simulink model "MyPCImages"  (Simulink 7.5)
settings: Solver=FixedStepDiscrete  StartTime=0.0  StopTime=d_data(end,1)  FixedStep=apSampleTime  RelTol=1e-3
InitFcn:
  | replayFlight
values from neighbouring files (symbols this model uses):
  apSampleTime = 0.01    [demoz2SlugsV5.m]
  D = y    [BarOrthog.m]
  R0 = single(Euler2DCMdeg( PHI_IC, THETA_IC, PSI_IC ))    [demoz2SlugsV5.m]
undefined symbols (not defined in the file or in its folder): accBiasRateLimit, accelXCutTemp, axTGain1, axTGain2, axTMean1, axTMean2, barAdjust, baroCutoff, baroCutTemp, baroOffset, baroScale, barTGain1, barTGain2, barTMean1, barTMean2, baseHeight, baseTemp, cubeAccelGain, cubeGyroGain, gaind, GS_location, gyroBiasRateLimit, Init_onlyOnce, Init_Reset, ISA_rho0, lapseRate, lowRateSensorCutoff, magMeanTemp, magOffset, magScale, magTempK, mainSensorCutoff, maxDynPressure, param_acc, param_mag, pitAdjust, pitCutTemp, pitotOffset, pitotScale, pitTGain1, pitTGain2, pitTMean1, pitTMean2, polesd, powerOffset, powerScale, pressureSensorCutoff, T, tempOffset, tempScale, vzCutoff, xCutoff, yCutoff, zCutoff, zerosd
libraries: simulink x11, aerolibconvert2 x9, SLUGS_Library x6, aerolibutil x3, dspmtrx3 x3, dsPICdrivers x1
(part 4 of 4)

== system MyPCImages/Sensor Data/Sensor Suite/Low Pass Filtering,Temperature Compensation and Calibration/Baro Altimeter/Zero Out Height ==
  Base Height : Inport  OutDataType=sfix(16)  OutScaling=2^0
  Computed Height : Inport  Port=2  OutDataType=sfix(16)  OutScaling=2^0
  Enable : EnablePort
  Integer Delay : simulink/Discrete/Integer Delay  vinit=0  samptime=.01  NumDelays=1
  Sum : Sum  Inputs=|+-  OutDataTypeMode=single  OutDataType=sfix(16)  OutScaling=2^0  OutDataTypeStr=single
  Height Offset : Outport  OutDataType=sfix(16)  OutScaling=2^0
  wires:
  Base Height/1 -> Sum/1
  Integer Delay/1 -> Sum/2
  Sum/1 -> Height Offset/1
  Computed Height/1 -> Integer Delay/1

== system MyPCImages/Sensor Data/Sensor Suite/Low Pass Filtering,Temperature Compensation and Calibration/Temp Compensate Accel X1/Hi Temp Compensation2 ==
  Raw : Inport  OutDataType=sfix(16)  OutScaling=2^0
  Temp Raw : Inport  Port=2  OutDataType=sfix(16)  OutScaling=2^0
  Enable : EnablePort
  Divide1 : Product  OutDataTypeMode=single  OutDataType=sfix(16)  OutScaling=2^-10  OutDataTypeStr=single
  Mean Temperature for Calibration : Constant  Value=tempMean  OutDataTypeMode=single  OutDataType=sfix(16)  OutScaling=2^0  OutDataTypeStr=single
  Sum1 : Sum  Inputs=|+-  OutDataTypeMode=single  OutDataType=sfix(16)  OutScaling=2^0  OutDataTypeStr=single
  Sum2 : Sum  Inputs=|+-  OutDataTypeMode=single  OutDataType=sfix(16)  OutScaling=2^0  OutDataTypeStr=single
  gains : Constant  Value=alpha  OutDataTypeMode=single  OutDataType=sfix(16)  OutScaling=2^0  OutDataTypeStr=single
  Comp : Outport  OutDataType=sfix(16)  OutScaling=2^0
  wires:
  Sum2/1 -> Comp/1
  Divide1/1 -> Sum2/2
  gains/1 -> Divide1/1
  Sum1/1 -> Divide1/2
  Temp Raw/1 -> Sum1/1
  Raw/1 -> Sum2/1
  Mean Temperature for Calibration/1 -> Sum1/2

== system MyPCImages/Sensor Data/Sensor Suite/Low Pass Filtering,Temperature Compensation and Calibration/Temp Compensate Accel X1/Lo Temp Compensation ==
  Raw : Inport  OutDataType=sfix(16)  OutScaling=2^0
  Temp Raw : Inport  Port=2  OutDataType=sfix(16)  OutScaling=2^0
  Enable : EnablePort
  Add : Sum  OutDataTypeMode=single  OutDataType=sfix(16)  OutScaling=2^-10  OutDataTypeStr=single
  Constant : Constant  Value=pitAdjust  OutDataTypeMode=single  OutDataType=sfix(16)  OutScaling=2^0  OutDataTypeStr=single
  Divide1 : Product  OutDataTypeMode=single  OutDataType=sfix(16)  OutScaling=2^-10  OutDataTypeStr=single
  Mean Temperature for Calibration : Constant  Value=tempMean  OutDataTypeMode=single  OutDataType=sfix(16)  OutScaling=2^0  OutDataTypeStr=single
  Sum1 : Sum  Inputs=|+-  OutDataTypeMode=single  OutDataType=sfix(16)  OutScaling=2^0  OutDataTypeStr=single
  Sum2 : Sum  Inputs=|+-  OutDataTypeMode=single  OutDataType=sfix(16)  OutScaling=2^0  OutDataTypeStr=single
  gains : Constant  Value=alpha  OutDataTypeMode=single  OutDataType=sfix(16)  OutScaling=2^0  OutDataTypeStr=single
  Comp : Outport  OutDataType=sfix(16)  OutScaling=2^0
  wires:
  Mean Temperature for Calibration/1 -> Sum1/2
  Raw/1 -> Sum2/1
  Temp Raw/1 -> Sum1/1
  Sum1/1 -> Divide1/2
  gains/1 -> Divide1/1
  Divide1/1 -> Sum2/2
  Sum2/1 -> Add/1
  Constant/1 -> Add/2
  Add/1 -> Comp/1

== system MyPCImages/Sensor Data/Sensor Suite/Low Pass Filtering,Temperature Compensation and Calibration/Temp Compensate Baro/Hi Temp Compensation ==
  Raw : Inport  OutDataType=sfix(16)  OutScaling=2^0
  Temp Raw : Inport  Port=2  OutDataType=sfix(16)  OutScaling=2^0
  Enable : EnablePort
  Add : Sum  OutDataTypeMode=single  OutDataType=sfix(16)  OutScaling=2^-10  OutDataTypeStr=single
  Constant : Constant  Value=barAdjust  OutDataTypeMode=single  OutDataType=sfix(16)  OutScaling=2^0  OutDataTypeStr=single
  Divide1 : Product  OutDataTypeMode=single  OutDataType=sfix(16)  OutScaling=2^-10  OutDataTypeStr=single
  Mean Temperature for Calibration : Constant  Value=tempMean  OutDataTypeMode=single  OutDataType=sfix(16)  OutScaling=2^0  OutDataTypeStr=single
  Sum1 : Sum  Inputs=|+-  OutDataTypeMode=single  OutDataType=sfix(16)  OutScaling=2^0  OutDataTypeStr=single
  Sum2 : Sum  Inputs=|+-  OutDataTypeMode=single  OutDataType=sfix(16)  OutScaling=2^0  OutDataTypeStr=single
  gains : Constant  Value=alpha  OutDataTypeMode=single  OutDataType=sfix(16)  OutScaling=2^0  OutDataTypeStr=single
  Comp : Outport  OutDataType=sfix(16)  OutScaling=2^0
  wires:
  Mean Temperature for Calibration/1 -> Sum1/2
  Raw/1 -> Sum2/1
  Temp Raw/1 -> Sum1/1
  Sum1/1 -> Divide1/2
  gains/1 -> Divide1/1
  Divide1/1 -> Sum2/2
  Constant/1 -> Add/1
  Add/1 -> Comp/1
  Sum2/1 -> Add/2

== system MyPCImages/Sensor Data/Sensor Suite/Low Pass Filtering,Temperature Compensation and Calibration/Temp Compensate Baro/Lo Temp Compensation ==
  Raw : Inport  OutDataType=sfix(16)  OutScaling=2^0
  Temp Raw : Inport  Port=2  OutDataType=sfix(16)  OutScaling=2^0
  Enable : EnablePort
  Divide1 : Product  OutDataTypeMode=single  OutDataType=sfix(16)  OutScaling=2^-10  OutDataTypeStr=single
  Mean Temperature for Calibration : Constant  Value=tempMean  OutDataTypeMode=single  OutDataType=sfix(16)  OutScaling=2^0  OutDataTypeStr=single
  Sum1 : Sum  Inputs=|+-  OutDataTypeMode=single  OutDataType=sfix(16)  OutScaling=2^0  OutDataTypeStr=single
  Sum2 : Sum  Inputs=|+-  OutDataTypeMode=single  OutDataType=sfix(16)  OutScaling=2^0  OutDataTypeStr=single
  gains : Constant  Value=alpha  OutDataTypeMode=single  OutDataType=sfix(16)  OutScaling=2^0  OutDataTypeStr=single
  Comp : Outport  OutDataType=sfix(16)  OutScaling=2^0
  wires:
  Sum2/1 -> Comp/1
  Divide1/1 -> Sum2/2
  gains/1 -> Divide1/1
  Sum1/1 -> Divide1/2
  Temp Raw/1 -> Sum1/1
  Raw/1 -> Sum2/1
  Mean Temperature for Calibration/1 -> Sum1/2

== system MyPCImages/Sensor Data/Sensor Suite/Low Pass Filtering,Temperature Compensation and Calibration/ValidateMags/Hold if Outlier ==
  In1 : Inport  OutDataType=sfix(16)  OutScaling=2^0
  Enable : EnablePort
  Out1 : Outport  OutDataType=sfix(16)  OutScaling=2^0  OutputWhenDisabled=reset  InitialOutput=[0 0 0]
  wires:
  In1/1 -> Out1/1

== system MyPCImages/Sensor Data/Sensor Suite/Low Pass Filtering,Temperature Compensation and Calibration/ValidateMags/Monitor Norm ==
  Mags : Inport  OutDataType=sfix(16)  OutScaling=2^0
  0.7 < Norm < 1.5 : Subsystem
  Norm : Subsystem  AncestorBlock=SLUGS_Library/Navigation/Norm
  Enable : Outport  OutDataType=sfix(16)  OutScaling=2^0
  wires:
  Mags/1 -> Norm/1(Vector)
  0.7 < Norm < 1.5/1(flag) -> Enable/1
  Norm/1(Norm) -> 0.7 < Norm < 1.5/1(norm)

== system MyPCImages/Position and Attitude Filter/Position Filter/BlendPosVel/2 FIlter Blend/1D Filter/Filter2 ==
  In1 : Inport  OutDataType=sfix(16)  OutScaling=2^0
  Discrete Zero-Pole : DiscreteZeroPole  Zeros=zerosd  Poles=polesd  Gain=gaind  SampleTime=SampleTime
  Out1 : Outport  OutDataType=sfix(16)  OutScaling=2^0
  wires:
  Discrete Zero-Pole/1 -> Out1/1
  In1/1 -> Discrete Zero-Pole/1

== system MyPCImages/Position and Attitude Filter/Position Filter/BlendPosVel/2 FIlter Blend/1D Filter1/Filter2 ==
  In1 : Inport  OutDataType=sfix(16)  OutScaling=2^0
  Discrete Zero-Pole : DiscreteZeroPole  Zeros=zerosd  Poles=polesd  Gain=gaind  SampleTime=SampleTime
  Out1 : Outport  OutDataType=sfix(16)  OutScaling=2^0
  wires:
  In1/1 -> Discrete Zero-Pole/1
  Discrete Zero-Pole/1 -> Out1/1

== system MyPCImages/Position and Attitude Filter/Position Filter/BlendPosVel/CompFiltRate/1D Filter1/Filter2 ==
  In1 : Inport  OutDataType=sfix(16)  OutScaling=2^0
  Discrete Zero-Pole : DiscreteZeroPole  Zeros=zerosd  Poles=polesd  Gain=gaind  SampleTime=SampleTime
  Out1 : Outport  OutDataType=sfix(16)  OutScaling=2^0
  wires:
  In1/1 -> Discrete Zero-Pole/1
  Discrete Zero-Pole/1 -> Out1/1

== system MyPCImages/Position and Attitude Filter/Position Filter/BlendPosVel/CompFiltRate1/1D Filter1/Filter2 ==
  In1 : Inport  OutDataType=sfix(16)  OutScaling=2^0
  Discrete Zero-Pole : DiscreteZeroPole  Zeros=zerosd  Poles=polesd  Gain=gaind  SampleTime=SampleTime
  Out1 : Outport  OutDataType=sfix(16)  OutScaling=2^0
  wires:
  In1/1 -> Discrete Zero-Pole/1
  Discrete Zero-Pole/1 -> Out1/1

== system MyPCImages/Position and Attitude Filter/Position Filter/BlendPosVel/CompRateOnly/1D Filter1/Filter2 ==
  In1 : Inport  OutDataType=sfix(16)  OutScaling=2^0
  Discrete Zero-Pole : DiscreteZeroPole  Zeros=zerosd  Poles=polesd  Gain=gaind  SampleTime=SampleTime
  Out1 : Outport  OutDataType=sfix(16)  OutScaling=2^0
  wires:
  In1/1 -> Discrete Zero-Pole/1
  Discrete Zero-Pole/1 -> Out1/1

== system MyPCImages/Sensor Data/Sensor Suite/Low Pass Filtering,Temperature Compensation and Calibration/Baro Altimeter/Initial Baro Bias/Low Pass8 ==
  In1 : Inport  OutDataType=sfix(16)  OutScaling=2^0
  Discrete Zero-Pole : DiscreteZeroPole  Zeros=zerosd  Poles=polesd  Gain=gaind  SampleTime=SampleTime
  Out1 : Outport  OutDataType=sfix(16)  OutScaling=2^0
  wires:
  Discrete Zero-Pole/1 -> Out1/1
  In1/1 -> Discrete Zero-Pole/1

== system MyPCImages/Sensor Data/Sensor Suite/Low Pass Filtering,Temperature Compensation and Calibration/ValidateMags/Monitor Norm/0.7 < Norm < 1.5 ==
  norm : Inport  OutDataType=sfix(16)  OutScaling=2^0
  Compare To Constant : simulink/Logic and Bit Operations/Compare To Constant  SystemSampleTime=-1  relop=>  const=0.5  LogicOutDataTypeMode=uint8  ZeroCross=off
  Compare To Constant1 : simulink/Logic and Bit Operations/Compare To Constant  SystemSampleTime=-1  relop=<  const=1.6  LogicOutDataTypeMode=uint8  ZeroCross=off
  Logical Operator : Logic  AllPortsSameDT=off  OutDataTypeMode=boolean  OutDataTypeStr=boolean
  flag : Outport  OutDataType=sfix(16)  OutScaling=2^0
  wires:
  Logical Operator/1 -> flag/1
  norm/1 -> Compare To Constant1/1, Compare To Constant/1
  Compare To Constant/1 -> Logical Operator/1
  Compare To Constant1/1 -> Logical Operator/2

== system MyPCImages/Sensor Data/Sensor Suite/Low Pass Filtering,Temperature Compensation and Calibration/ValidateMags/Monitor Norm/Norm ==
  Vector : Inport  OutDataType=sfix(16)  OutScaling=2^0
  Subsystem1 : Subsystem  AncestorBlock=SLUGS_Library/Subsystem1
  Subsystem3 : Subsystem  AncestorBlock=SLUGS_Library/Subsystem3
  Norm : Outport  OutDataType=sfix(16)  OutScaling=2^0
  wires:
  Subsystem3/1(x dot y) -> Subsystem1/1(x)
  Vector/1 -> Subsystem3/2(y), Subsystem3/1(x)
  Subsystem1/1(sqrt(x)) -> Norm/1

== system MyPCImages/Sensor Data/Sensor Suite/Low Pass Filtering,Temperature Compensation and Calibration/ValidateMags/Monitor Norm/Norm/Subsystem1 ==
  x : Inport  OutDataType=sfix(16)  OutScaling=2^0
  C Function Call : dsPICdrivers/OTHERS/C Function Call  Tag=dsPIC_dsPIC_CFunctionCall  FctUpdate=Output Function  fctName='mySqrt'  INPUT_SIZE=1  INPUT1=real32  INPUT2=--  INPUT3=--  OUTPUT_SIZE=1  OUTPUT1=real32  SampleTime=-1  InputType=[ 7 ]  OutputType=[ 7 ]  FctDeclaration=extern real32_T mySqrt(real32_T u1);  FctCall=%y1 = mySqrt(%u1);  OrderingInOutPopup=None  FctStart=None  FctStart_Name=Init_onlyOnce  FctStart_Declaration=inline extern void Init_onlyOnce();  FctStart_Call=Init_onlyOnce();  FctInit=None  FctInit_Name=Init_Reset  FctInit_Declaration=inline extern void Init_Reset();  FctInit_Call=Init_Reset();  PinDigitalInput=[]  PinDigitalOutput=[]  AnalogueInput=[]
  negprotect : Stateflow chart  TreatAsAtomicUnit=on
  sqrt(x) : Outport  OutDataType=sfix(16)  OutScaling=2^0
  wires:
  C Function Call/1 -> sqrt(x)/1
  negprotect/1(zpVal) -> C Function Call/1
  x/1 -> negprotect/1(val)

== system MyPCImages/Sensor Data/Sensor Suite/Low Pass Filtering,Temperature Compensation and Calibration/ValidateMags/Monitor Norm/Norm/Subsystem3 ==
  x : Inport  OutDataType=sfix(16)  OutScaling=2^0
  y : Inport  Port=2  OutDataType=sfix(16)  OutScaling=2^0
  Embedded MATLAB Function : Stateflow chart  TreatAsAtomicUnit=on
  x dot y : Outport  OutDataType=sfix(16)  OutScaling=2^0
  wires:
  y/1 -> Embedded MATLAB Function/2(y)
  x/1 -> Embedded MATLAB Function/1(x)
  Embedded MATLAB Function/1(xDoty) -> x dot y/1

== matlab function Sensor Data/Sensor Suite/Low Pass Filtering,Temperature Compensation and Calibration/Tustin Lowpass, Auto Initial Condition2/Embedded MATLAB Function ==
  data: u input double; y output double; T input double; f input double
function y = fcn(u,T,f)
% This block supports an embeddable subset of the MATLAB language.
% See the help menu for details. 

persistent a
persistent b
persistent y_km1
persistent u_km1
if isempty(a)
    %tf = [T*omega/(2+T*omega) T*omega/(2+T*omega)],[1 (T*omega-2)/(T*omega+2)]
    %tf = [a a],[1 -b]
    omega = 2*pi*f;
    a=T*omega/(2+T*omega);
    b=-(T*omega-2)/(T*omega+2);
    y_km1=u;
    u_km1=u;
end

y = a*(u+u_km1)+b*y_km1;
y_km1=y;
u_km1=u;

== matlab function Sensor Data/Sensor Suite/Low Pass Filtering,Temperature Compensation and Calibration/Tustin Lowpass, Auto Initial Condition3/Embedded MATLAB Function ==
  data: u input double; y output double; T input double; f input double
function y = fcn(u,T,f)
% This block supports an embeddable subset of the MATLAB language.
% See the help menu for details. 

persistent a
persistent b
persistent y_km1
persistent u_km1
if isempty(a)
    %tf = [T*omega/(2+T*omega) T*omega/(2+T*omega)],[1 (T*omega-2)/(T*omega+2)]
    %tf = [a a],[1 -b]
    omega = 2*pi*f;
    a=T*omega/(2+T*omega);
    b=-(T*omega-2)/(T*omega+2);
    y_km1=u;
    u_km1=u;
end

y = a*(u+u_km1)+b*y_km1;
y_km1=y;
u_km1=u;

== matlab function Sensor Data/Sensor Suite/Low Pass Filtering,Temperature Compensation and Calibration/3D Tustin Lowpass, Auto Initial Condition/Embedded MATLAB Function ==
  data: u input double; y output double; T input double; f input double
function y = fcn(u,T,f)
% This block supports an embeddable subset of the MATLAB language.
% See the help menu for details. 

persistent a
persistent b
persistent y_km1
persistent u_km1
if isempty(a)
    %tf = [T*omega/(2+T*omega) T*omega/(2+T*omega)],[1 (T*omega-2)/(T*omega+2)]
    %tf = [a a],[1 -b]
    omega = 2*pi*f;
    a=T*omega/(2+T*omega);
    b=-(T*omega-2)/(T*omega+2);
    y_km1=u;
    u_km1=u;
end

y = a*(u+u_km1)+b*y_km1;
y_km1=y;
u_km1=u;

== matlab function Sensor Data/Sensor Suite/Low Pass Filtering,Temperature Compensation and Calibration/3D Tustin Lowpass, Auto Initial Condition/Embedded MATLAB Function1 ==
  data: u input double; y output double; T input double; f input double
function y = fcn(u,T,f)
% This block supports an embeddable subset of the MATLAB language.
% See the help menu for details. 

persistent a
persistent b
persistent y_km1
persistent u_km1
if isempty(a)
    %tf = [T*omega/(2+T*omega) T*omega/(2+T*omega)],[1 (T*omega-2)/(T*omega+2)]
    %tf = [a a],[1 -b]
    omega = 2*pi*f;
    a=T*omega/(2+T*omega);
    b=-(T*omega-2)/(T*omega+2);
    y_km1=u;
    u_km1=u;
end

y = a*(u+u_km1)+b*y_km1;
y_km1=y;
u_km1=u;

== matlab function Sensor Data/Sensor Suite/Low Pass Filtering,Temperature Compensation and Calibration/3D Tustin Lowpass, Auto Initial Condition/myMux Fun ==
  data: u1 input double; y output double; u2 input double; u3 input double
function y = myMux3(u1, u2, u3)
% This block supports an embeddable subset of the MATLAB language.
% See the help menu for details. 

y = [u1(1); u2(1); u3(1)];

== matlab function Sensor Data/Sensor Suite/Low Pass Filtering,Temperature Compensation and Calibration/Tustin Lowpass, Auto Initial Condition4/Embedded MATLAB Function ==
  data: u input double; y output double; T input double; f input double
function y = fcn(u,T,f)
% This block supports an embeddable subset of the MATLAB language.
% See the help menu for details. 

persistent a
persistent b
persistent y_km1
persistent u_km1
if isempty(a)
    %tf = [T*omega/(2+T*omega) T*omega/(2+T*omega)],[1 (T*omega-2)/(T*omega+2)]
    %tf = [a a],[1 -b]
    omega = 2*pi*f;
    a=T*omega/(2+T*omega);
    b=-(T*omega-2)/(T*omega+2);
    y_km1=u;
    u_km1=u;
end

y = a*(u+u_km1)+b*y_km1;
y_km1=y;
u_km1=u;

== matlab function Position and Attitude Filter/Attitude Complimentary Filter COG/3D Filter/myMux Fun1 ==
  data: u1 input double; y output double; u2 input double; u3 input double
function y = myMux(u1, u2, u3)
% This block supports an embeddable subset of the MATLAB language.
% See the help menu for details. 

y = [u1(1); u2(1); u3(1)];

== matlab function Sensor Data/Sensor Suite/Low Pass Filtering,Temperature Compensation and Calibration/Baro Altimeter/Enables/Disables the Computation of initial Baro Bias ==
  data: tOut output double
function tOut = getTIni

persistent aveCount;
persistent tIni;

if isempty(aveCount)
    aveCount =1;
    tIni = 1;
end;

if aveCount < 2500
    aveCount = aveCount + 1;
end

if aveCount == 2500
    tIni =0;
    aveCount = aveCount + 1;
end

tOut = tIni;

%if aveCount > 500
%    tIni = 0;
%end

% if isempty(aveCount)
%     aveCount =1;
%     initBias = [0.0 0.0 0.0]';
% end;
%     
% if (aveCount<10)
%     initBias = initBias+ Raw;
%     bias = initBias/aveCount;
%     aveCount = aveCount +1;
% end;
% 
% if (aveCount == 10)
%     initBias = initBias/(aveCount-1);
%     aveCount = 100;
% end;
% 
% if (aveCount == 100)
%     bias = initBias;
% end;

== matlab function Position and Attitude Filter/Attitude Complimentary Filter COG/Embedded MATLAB Function ==
  data: u input double; y output double
function y = TwoPi(u)
% This block supports an embeddable subset of the MATLAB language.
% See the help menu for details. 

if ( u < 0 )
    y = u + 2*pi;
else
    y = u;
end

== matlab function Sensor Data/Sensor Suite/Low Pass Filtering,Temperature Compensation and Calibration/3D Tustin Lowpass, Auto Initial Condition/Embedded MATLAB Function2 ==
  data: u input double; y output double; T input double; f input double
function y = fcn(u,T,f)
% This block supports an embeddable subset of the MATLAB language.
% See the help menu for details. 

persistent a
persistent b
persistent y_km1
persistent u_km1
if isempty(a)
    %tf = [T*omega/(2+T*omega) T*omega/(2+T*omega)],[1 (T*omega-2)/(T*omega+2)]
    %tf = [a a],[1 -b]
    omega = 2*pi*f;
    a=T*omega/(2+T*omega);
    b=-(T*omega-2)/(T*omega+2);
    y_km1=u;
    u_km1=u;
end

y = a*(u+u_km1)+b*y_km1;
y_km1=y;
u_km1=u;

== matlab function Sensor Data/Sensor Suite/Cube Signal Cond/3D Tustin Lowpass, Auto Initial Condition/Embedded MATLAB Function ==
  data: u input double; y output double; T input double; f input double
function y = fcn(u,T,f)
% This block supports an embeddable subset of the MATLAB language.
% See the help menu for details. 

persistent a
persistent b
persistent y_km1
persistent u_km1
if isempty(a)
    %tf = [T*omega/(2+T*omega) T*omega/(2+T*omega)],[1 (T*omega-2)/(T*omega+2)]
    %tf = [a a],[1 -b]
    omega = 2*pi*f;
    a=T*omega/(2+T*omega);
    b=-(T*omega-2)/(T*omega+2);
    y_km1=u;
    u_km1=u;
end

y = a*(u+u_km1)+b*y_km1;
y_km1=y;
u_km1=u;

== matlab function Sensor Data/Sensor Suite/Low Pass Filtering,Temperature Compensation and Calibration/Tustin Lowpass, Auto Initial Condition1/Embedded MATLAB Function ==
  data: u input double; y output double; T input double; f input double
function y = fcn(u,T,f)
% This block supports an embeddable subset of the MATLAB language.
% See the help menu for details. 

persistent a
persistent b
persistent y_km1
persistent u_km1
if isempty(a)
    %tf = [T*omega/(2+T*omega) T*omega/(2+T*omega)],[1 (T*omega-2)/(T*omega+2)]
    %tf = [a a],[1 -b]
    omega = 2*pi*f;
    a=T*omega/(2+T*omega);
    b=-(T*omega-2)/(T*omega+2);
    y_km1=u;
    u_km1=u;
end

y = a*(u+u_km1)+b*y_km1;
y_km1=y;
u_km1=u;

== matlab function Position and Attitude Filter/Attitude Complimentary Filter COG/myMux Fun1 ==
  data: u1 input double; y output double; u2 input double; u3 input double
function y = myMux3(u1, u2, u3)
% This block supports an embeddable subset of the MATLAB language.
% See the help menu for details. 

y = [u1(1); u2(1); u3(1)];

== matlab function Sensor Data/Sensor Suite/Low Pass Filtering,Temperature Compensation and Calibration/ValidateMags/Monitor Norm/Norm/Subsystem3/Embedded MATLAB Function ==
  data: x input double; y input double; xDoty output double
function xDoty = myDot(x,y)
% This block supports an embeddable subset of the MATLAB language.
% See the help menu for details. 

xDoty = x(1)*y(1) + x(2)*y(2) + x(3)*y(3);

== matlab function Sensor Data/Sensor Suite/Cube Signal Cond/3D Tustin Lowpass, Auto Initial Condition/Embedded MATLAB Function1 ==
  data: u input double; y output double; T input double; f input double
function y = fcn(u,T,f)
% This block supports an embeddable subset of the MATLAB language.
% See the help menu for details. 

persistent a
persistent b
persistent y_km1
persistent u_km1
if isempty(a)
    %tf = [T*omega/(2+T*omega) T*omega/(2+T*omega)],[1 (T*omega-2)/(T*omega+2)]
    %tf = [a a],[1 -b]
    omega = 2*pi*f;
    a=T*omega/(2+T*omega);
    b=-(T*omega-2)/(T*omega+2);
    y_km1=u;
    u_km1=u;
end

y = a*(u+u_km1)+b*y_km1;
y_km1=y;
u_km1=u;

== matlab function Sensor Data/Sensor Suite/Low Pass Filtering,Temperature Compensation and Calibration/ValidateMags/Monitor Norm/Norm/Subsystem1/negprotect ==
  data: val input double; zpVal output double
function zpVal = negProt(val)
% This block supports an embeddable subset of the MATLAB language.
% See the help menu for details. 

if val >= single(0.001)
    zpVal = val;
else
    zpVal = single(0.001);
end

== matlab function Position and Attitude Filter/Position Filter/BlendPosVel/3D Filter/myMux Fun1 ==
  data: u1 input double; y output double; u2 input double; u3 input double
function y = myMux(u1, u2, u3)
% This block supports an embeddable subset of the MATLAB language.
% See the help menu for details. 

y = [u1(1); u2(1); u3(1)];

== matlab function Sensor Data/Sensor Suite/Cube Signal Cond/3D Tustin Lowpass, Auto Initial Condition/Embedded MATLAB Function2 ==
  data: u input double; y output double; T input double; f input double
function y = fcn(u,T,f)
% This block supports an embeddable subset of the MATLAB language.
% See the help menu for details. 

persistent a
persistent b
persistent y_km1
persistent u_km1
if isempty(a)
    %tf = [T*omega/(2+T*omega) T*omega/(2+T*omega)],[1 (T*omega-2)/(T*omega+2)]
    %tf = [a a],[1 -b]
    omega = 2*pi*f;
    a=T*omega/(2+T*omega);
    b=-(T*omega-2)/(T*omega+2);
    y_km1=u;
    u_km1=u;
end

y = a*(u+u_km1)+b*y_km1;
y_km1=y;
u_km1=u;

== matlab function Sensor Data/Sensor Suite/If no HIL then Read all the Sensors/myMux Fun4 ==
  data: u1 input double; y output double; u2 input double; u3 input double; u4 input double; u5 input double; u6 input double; u7 input double; u8 input double; u9 input double; u10 input double; u11 input double; u12 input double; u13 input double
function y = sensMux(u1, u2,u3,u4,u5,u6,u7,u8, u9, u10, u11, u12, u13)
% This block supports an embeddable subset of the MATLAB language.
% See the help menu for details. 

y = [u1(1); u2(1); u3(1); u4(1); u5(1); u6(1); u7(1); u8(1); u9(1); u10(1); u11(1); u12(1); u13(1)];

== matlab function Sensor Data/Sensor Suite/Cube Signal Cond/3D Tustin Lowpass, Auto Initial Condition/myMux Fun ==
  data: u1 input double; y output double; u2 input double; u3 input double
function y = myMux3(u1, u2, u3)
% This block supports an embeddable subset of the MATLAB language.
% See the help menu for details. 

y = [u1(1); u2(1); u3(1)];

== matlab function Sensor Data/Sensor Suite/Low Pass Filtering,Temperature Compensation and Calibration/Ellipse Correction/myMux Fun3 ==
  data: u1 input double; y output double; u2 input double; u3 input double
function y = myMux(u1, u2, u3)
% This block supports an embeddable subset of the MATLAB language.
% See the help menu for details. 

y = [u1(1); u2(1); u3(1)];

== matlab function Sensor Data/Sensor Suite/Cube Signal Cond/Ellipse Correction/myMux Fun3 ==
  data: u1 input double; y output double; u2 input double; u3 input double
function y = myMux(u1, u2, u3)
% This block supports an embeddable subset of the MATLAB language.
% See the help menu for details. 

y = [u1(1); u2(1); u3(1)];

== matlab function Position and Attitude Filter/Position Filter/BlendPosVel/Embedded MATLAB Function1 ==
  data: u input double size=1; y output double size=1; NewGPS input double size=1; apSampleTime parameter double size=1
function y = RateAid(u,NewGPS,apSampleTime)
persistent LastU;
persistent TimeSinceLast;
persistent NGPS;
persistent rate;
persistent OldRate;

if (isempty(LastU))
    LastU = single(0.);
    TimeSinceLast = single(0);
    NGPS = single(0);
    rate = single(0);
    OldRate = single(0);
end

if (NewGPS)
    if ( NGPS ~= 0 )
        OldRate = rate;
        rate = single((u - LastU)/TimeSinceLast);
        TimeSinceLast = single(0);
        LastU = u;
    else
        rate = single(0);
        OldRate = single(0);
    end
    NGPS = NGPS + 1;
end
y = u + ( .5*rate + .5*OldRate )*TimeSinceLast;
TimeSinceLast = TimeSinceLast + apSampleTime;

== matlab function Sensor Data/Sensor Suite/Cube Signal Cond/3D Tustin Lowpass, Auto Initial Condition1/Embedded MATLAB Function ==
  data: u input double; y output double; T input double; f input double
function y = fcn(u,T,f)
% This block supports an embeddable subset of the MATLAB language.
% See the help menu for details. 

persistent a
persistent b
persistent y_km1
persistent u_km1
if isempty(a)
    %tf = [T*omega/(2+T*omega) T*omega/(2+T*omega)],[1 (T*omega-2)/(T*omega+2)]
    %tf = [a a],[1 -b]
    omega = 2*pi*f;
    a=T*omega/(2+T*omega);
    b=-(T*omega-2)/(T*omega+2);
    y_km1=u;
    u_km1=u;
end

y = a*(u+u_km1)+b*y_km1;
y_km1=y;
u_km1=u;

== matlab function Sensor Data/Sensor Suite/Cube Signal Cond/3D Tustin Lowpass, Auto Initial Condition1/Embedded MATLAB Function1 ==
  data: u input double; y output double; T input double; f input double
function y = fcn(u,T,f)
% This block supports an embeddable subset of the MATLAB language.
% See the help menu for details. 

persistent a
persistent b
persistent y_km1
persistent u_km1
if isempty(a)
    %tf = [T*omega/(2+T*omega) T*omega/(2+T*omega)],[1 (T*omega-2)/(T*omega+2)]
    %tf = [a a],[1 -b]
    omega = 2*pi*f;
    a=T*omega/(2+T*omega);
    b=-(T*omega-2)/(T*omega+2);
    y_km1=u;
    u_km1=u;
end

y = a*(u+u_km1)+b*y_km1;
y_km1=y;
u_km1=u;

== matlab function Sensor Data/Sensor Suite/Cube Signal Cond/3D Tustin Lowpass, Auto Initial Condition1/Embedded MATLAB Function2 ==
  data: u input double; y output double; T input double; f input double
function y = fcn(u,T,f)
% This block supports an embeddable subset of the MATLAB language.
% See the help menu for details. 

persistent a
persistent b
persistent y_km1
persistent u_km1
if isempty(a)
    %tf = [T*omega/(2+T*omega) T*omega/(2+T*omega)],[1 (T*omega-2)/(T*omega+2)]
    %tf = [a a],[1 -b]
    omega = 2*pi*f;
    a=T*omega/(2+T*omega);
    b=-(T*omega-2)/(T*omega+2);
    y_km1=u;
    u_km1=u;
end

y = a*(u+u_km1)+b*y_km1;
y_km1=y;
u_km1=u;

== matlab function Sensor Data/Sensor Suite/Cube Signal Cond/3D Tustin Lowpass, Auto Initial Condition1/myMux Fun ==
  data: u1 input double; y output double; u2 input double; u3 input double
function y = myMux3(u1, u2, u3)
% This block supports an embeddable subset of the MATLAB language.
% See the help menu for details. 

y = [u1(1); u2(1); u3(1)];

== matlab function Position and Attitude Filter/Attitude Complimentary Filter COG/3D Filter2/myMux Fun1 ==
  data: u1 input double; y output double; u2 input double; u3 input double
function y = myMux(u1, u2, u3)
% This block supports an embeddable subset of the MATLAB language.
% See the help menu for details. 

y = [u1(1); u2(1); u3(1)];

== matlab function Position and Attitude Filter/COG.SOG2V/myMux Fun2 ==
  data: u1 input double; y output double; u2 input double; u3 input double
function y = myMux3(u1, u2, u3)
% This block supports an embeddable subset of the MATLAB language.
% See the help menu for details. 

y = [u1(1); u2(1); u3(1)];

== matlab function Position and Attitude Filter/Attitude Complimentary Filter COG/myMux Fun2 ==
  data: u1 input double; y output double; u2 input double; u3 input double
function y = myMux3(u1, u2, u3)
% This block supports an embeddable subset of the MATLAB language.
% See the help menu for details. 

y = [u1(1); u2(1); u3(1)];

== matlab function Position and Attitude Filter/Position Filter/BlendPosVel/myMux Fun1 ==
  data: u1 input double; y output double; u2 input double; u3 input double
function y = myMux3(u1, u2, u3)
% This block supports an embeddable subset of the MATLAB language.
% See the help menu for details. 

y = [u1(1); u2(1); u3(1)];

== matlab function Position and Attitude Filter/Position Filter/BlendPosVel/myMux Fun2 ==
  data: u1 input double; y output double; u2 input double; u3 input double
function y = myMux3(u1, u2, u3)
% This block supports an embeddable subset of the MATLAB language.
% See the help menu for details. 

y = [u1(1); u2(1); u3(1)];

== matlab function Position and Attitude Filter/Position Filter/BlendPosVel/myMux Fun3 ==
  data: u1 input double; y output double; u2 input double; u3 input double
function y = myMux3(u1, u2, u3)
% This block supports an embeddable subset of the MATLAB language.
% See the help menu for details. 

y = [u1(1); u2(1); u3(1)];

== matlab function Sensor Data/Sensor Suite/Cube Signal Cond/myMux Fun ==
  data: u1 input double; y output double; u2 input double; u3 input double
function y = myMux3(u1, u2, u3)
% This block supports an embeddable subset of the MATLAB language.
% See the help menu for details. 

y = [u1(1); u2(1); u3(1)];
